simulink model "sampleModel2403_pp_1_1_difftest_difftest"  (R2018a)
settings: Solver=VariableStepAuto  StartTime=0.0  StopTime=10.0  RelTol=1e-3
undefined symbols (not defined in the file): DiscIntNeverNeededParam, sigbuilder_block
libraries: simulink x106
(part 2 of 2)

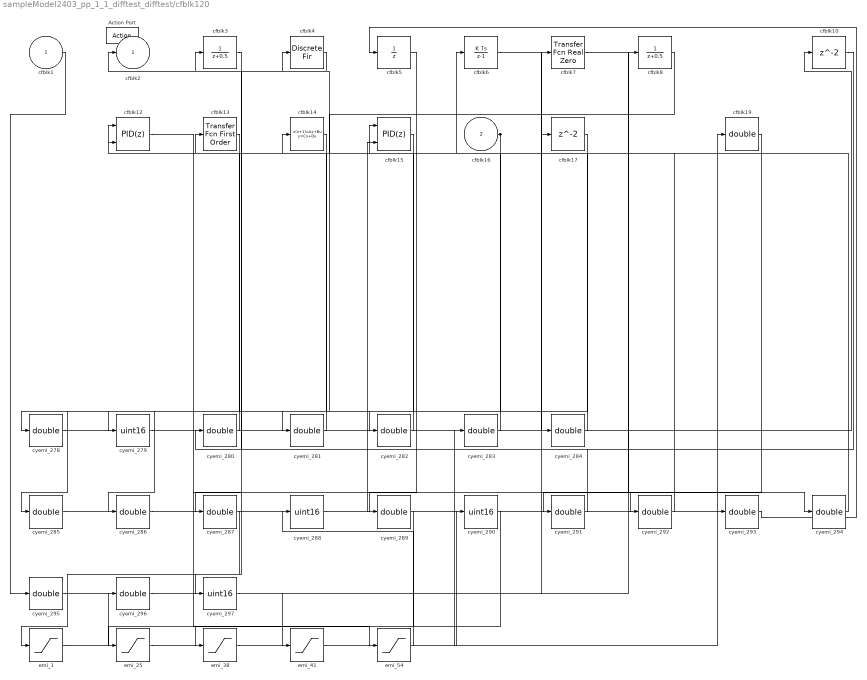
== system sampleModel2403_pp_1_1_difftest_difftest/cfblk120 ==
  cfblk1 : Inport
  cfblk16 : Inport  Port=2
  Action Port : ActionPort  ActionType=then
  cfblk10 : Delay
  cfblk12 : simulink/Continuous/PID Controller (2DOF)  Controller=PID  TimeDomain=Discrete-time  SampleTime=-1  IntegratorMethod=Forward Euler  FilterMethod=Forward Euler  Form=Parallel  UseFilter=on  ControllerParametersSource=internal  P=1  I=1  D=0  N=100  b=1  c=1  InitialConditionSource=internal  InitialConditionForIntegrator=0  InitialConditionForFilter=0  ExternalReset=none  LimitOutput=off  UpperSaturationLimit=inf  LowerSaturationLimit=-inf  LinearizeAsGain=off  AntiWindupMode=none  Kb=1  TrackingMode=off  Kt=1  PParamMin=[]  PParamMax=[]  IParamMin=[]  IParamMax=[]  DParamMin=[]  DParamMax=[]  NParamMin=[]  NParamMax=[]  bParamMin=[]  bParamMax=[]  cParamMin=[]  cParamMax=[]  KbParamMin=[]  KbParamMax=[]  KtParamMin=[]  KtParamMax=[]  POutMin=[]  POutMax=[]  IOutMin=[]  IOutMax=[]  DOutMin=[]  DOutMax=[]  NOutMin=[]  NOutMax=[]  bOutMin=[]  bOutMax=[]  cOutMin=[]  cOutMax=[]  KbOutMin=[]  KbOutMax=[]  KtOutMin=[]  KtOutMax=[]  IntegratorOutMin=[]  IntegratorOutMax=[]  FilterOutMin=[]  FilterOutMax=[]  SumOutMin=[]  SumOutMax=[]  Sum1OutMin=[]  Sum1OutMax=[]  Sum2OutMin=[]  Sum2OutMax=[]  Sum3OutMin=[]  Sum3OutMax=[]  SumI1OutMin=[]  SumI1OutMax=[]  SumI2OutMin=[]  SumI2OutMax=[]  SumI3OutMin=[]  SumI3OutMax=[]  SumDOutMin=[]  SumDOutMax=[]  SaturationOutMin=[]  SaturationOutMax=[]  IntegratorContinuousStateAttributes=''  IntegratorStateMustResolveToSignalObject=off  IntegratorRTWStateStorageClass=Auto  FilterContinuousStateAttributes=''  FilterStateMustResolveToSignalObject=off  FilterRTWStateStorageClass=Auto  DifferentiatorICPrevScaledInput=0  DifferentiatorOutMin=[]  DifferentiatorOutMax=[]  FilterDiffOutCoefMin=[]  FilterDiffOutCoefMax=[]  SumDenOutMin=[]  SumDenOutMax=[]  SumNumOutMin=[]  SumNumOutMax=[]  ReciprocalOutMin=[]  ReciprocalOutMax=[]  DivideOutMin=[]  DivideOutMax=[]  TunerSelectOption=Transfer Function Based (PID Tuner App)
  cfblk13 : simulink/Discrete/Transfer Fcn First Order  PoleZ=0.95  ICPrevOutput=0.0  DoSatur=off
      settings: SourceProductName=Simulink
  cfblk14 : DiscreteStateSpace  SampleTime=-1
  cfblk15 : simulink/Continuous/PID Controller (2DOF)  Controller=PID  TimeDomain=Discrete-time  SampleTime=-1  IntegratorMethod=Forward Euler  FilterMethod=Forward Euler  Form=Parallel  UseFilter=on  ControllerParametersSource=internal  P=1  I=1  D=0  N=100  b=1  c=1  InitialConditionSource=internal  InitialConditionForIntegrator=0  InitialConditionForFilter=0  ExternalReset=none  LimitOutput=off  UpperSaturationLimit=inf  LowerSaturationLimit=-inf  LinearizeAsGain=off  AntiWindupMode=none  Kb=1  TrackingMode=off  Kt=1  PParamMin=[]  PParamMax=[]  IParamMin=[]  IParamMax=[]  DParamMin=[]  DParamMax=[]  NParamMin=[]  NParamMax=[]  bParamMin=[]  bParamMax=[]  cParamMin=[]  cParamMax=[]  KbParamMin=[]  KbParamMax=[]  KtParamMin=[]  KtParamMax=[]  POutMin=[]  POutMax=[]  IOutMin=[]  IOutMax=[]  DOutMin=[]  DOutMax=[]  NOutMin=[]  NOutMax=[]  bOutMin=[]  bOutMax=[]  cOutMin=[]  cOutMax=[]  KbOutMin=[]  KbOutMax=[]  KtOutMin=[]  KtOutMax=[]  IntegratorOutMin=[]  IntegratorOutMax=[]  FilterOutMin=[]  FilterOutMax=[]  SumOutMin=[]  SumOutMax=[]  Sum1OutMin=[]  Sum1OutMax=[]  Sum2OutMin=[]  Sum2OutMax=[]  Sum3OutMin=[]  Sum3OutMax=[]  SumI1OutMin=[]  SumI1OutMax=[]  SumI2OutMin=[]  SumI2OutMax=[]  SumI3OutMin=[]  SumI3OutMax=[]  SumDOutMin=[]  SumDOutMax=[]  SaturationOutMin=[]  SaturationOutMax=[]  IntegratorContinuousStateAttributes=''  IntegratorStateMustResolveToSignalObject=off  IntegratorRTWStateStorageClass=Auto  FilterContinuousStateAttributes=''  FilterStateMustResolveToSignalObject=off  FilterRTWStateStorageClass=Auto  DifferentiatorICPrevScaledInput=0  DifferentiatorOutMin=[]  DifferentiatorOutMax=[]  FilterDiffOutCoefMin=[]  FilterDiffOutCoefMax=[]  SumDenOutMin=[]  SumDenOutMax=[]  SumNumOutMin=[]  SumNumOutMax=[]  ReciprocalOutMin=[]  ReciprocalOutMax=[]  DivideOutMin=[]  DivideOutMax=[]  TunerSelectOption=Transfer Function Based (PID Tuner App)
  cfblk17 : Delay
  cfblk19 : DataTypeConversion  OutDataTypeStr=double
  cfblk3 : DiscreteTransferFcn
  cfblk4 : DiscreteFir
  cfblk5 : UnitDelay  SampleTime=-1
  cfblk6 : DiscreteIntegrator  SampleTime=-1  OutDataTypeStr=double  ICPrevOutput=DiscIntNeverNeededParam  ICPrevScaledInput=DiscIntNeverNeededParam
  cfblk7 : simulink/Discrete/Transfer Fcn Real Zero  ZeroZ=0.75  ICPrevInput=0.0  DoSatur=off
      settings: SourceProductName=Simulink  SourceProductBaseCode=SL
  cfblk8 : DiscreteTransferFcn
  cyemi_{278,280..287,289,291..296} (16 alike) : DataTypeConversion  OutDataTypeStr=double
  cyemi_{279,288,290,297} (4 alike) : DataTypeConversion  OutDataTypeStr=uint16
  emi_{1,25,38,41,54} (5 alike) : Saturate  UpperLimit=0  LowerLimit=0
  cfblk2 : Outport
  wires:
  cfblk4/1 -> cfblk2/1
  cfblk16/1 -> cyemi_279/1, cyemi_297/1
  cyemi_278/1 -> cfblk10/1
  cfblk14/1 -> cyemi_278/1
  cyemi_280/1 -> cfblk12/1
  cfblk10/1 -> cyemi_280/1
  cyemi_281/1 -> cfblk12/2
  cfblk8/1 -> cyemi_281/1
  cyemi_282/1 -> cfblk13/1
  cfblk15/1 -> cyemi_282/1
  cyemi_283/1 -> cfblk14/1
  cyemi_284/1 -> cfblk15/1
  cfblk6/1 -> cyemi_284/1
  cyemi_285/1 -> cfblk15/2
  cfblk17/1 -> cyemi_285/1
  cyemi_286/1 -> cfblk17/1
  cfblk13/1 -> cyemi_286/1
  cfblk3/1 -> cyemi_287/1
  cyemi_288/1 -> cfblk19/1
  cfblk5/1 -> cyemi_289/1
  cyemi_291/1 -> cfblk3/1
  cfblk19/1 -> cyemi_291/1
  cyemi_292/1 -> cfblk4/1
  cfblk12/1 -> cyemi_292/1
  cyemi_293/1 -> cfblk5/1
  cyemi_294/1 -> cfblk6/1
  cfblk7/1 -> cyemi_294/1
  cyemi_295/1 -> cfblk7/1
  cfblk1/1 -> cyemi_295/1
  cyemi_296/1 -> cfblk8/1
  emi_1/1 -> cyemi_296/1
  cyemi_287/1 -> emi_1/1
  emi_25/1 -> cyemi_293/1
  cyemi_290/1 -> emi_25/1
  emi_38/1 -> cyemi_283/1
  cyemi_289/1 -> emi_38/1
  emi_41/1 -> cyemi_290/1
  cyemi_297/1 -> emi_41/1
  emi_54/1 -> cyemi_288/1
  cyemi_279/1 -> emi_54/1

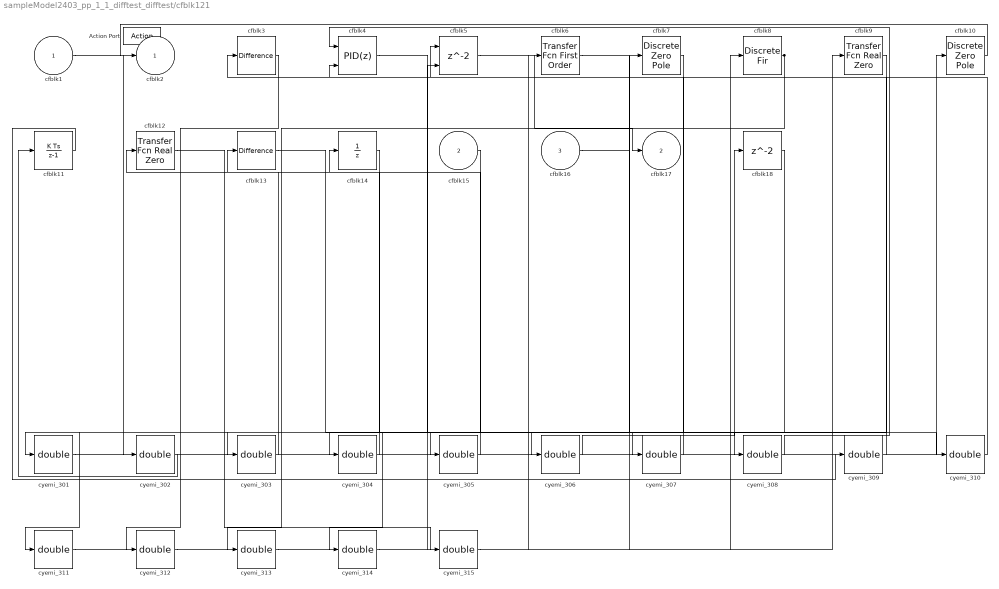
== system sampleModel2403_pp_1_1_difftest_difftest/cfblk121 ==
  cfblk1 : Inport
  cfblk15 : Inport  Port=2
  cfblk16 : Inport  Port=3
  Action Port : ActionPort  ActionType=else
  cfblk10 : DiscreteZeroPole  Poles=[0 0.5]  Gain=1  SampleTime=-1
  cfblk11 : DiscreteIntegrator  SampleTime=-1  OutDataTypeStr=double  ICPrevOutput=DiscIntNeverNeededParam  ICPrevScaledInput=DiscIntNeverNeededParam
  cfblk12 : simulink/Discrete/Transfer Fcn Real Zero  ZeroZ=0.75  ICPrevInput=0.0  DoSatur=off
      settings: SourceProductName=Simulink  SourceProductBaseCode=SL
  cfblk13 : simulink/Discrete/Difference  ICPrevInput=0.0  OutMin=[]  OutMax=[]  OutDataTypeStr=double  OutputDataTypeScalingMode=double  OutDataType=fixdt(1, 16)  OutScaling=2^-10  DoSatur=off
  cfblk14 : UnitDelay  SampleTime=-1
  cfblk18 : Delay
  cfblk3 : simulink/Discrete/Difference  ICPrevInput=0.0  OutMin=[]  OutMax=[]  OutDataTypeStr=double  OutputDataTypeScalingMode=double  OutDataType=fixdt(1, 16)  OutScaling=2^-10  DoSatur=off
  cfblk4 : simulink/Continuous/PID Controller (2DOF)  Controller=PID  TimeDomain=Discrete-time  SampleTime=-1  IntegratorMethod=Forward Euler  FilterMethod=Forward Euler  Form=Parallel  UseFilter=on  ControllerParametersSource=internal  P=1  I=1  D=0  N=100  b=1  c=1  InitialConditionSource=internal  InitialConditionForIntegrator=0  InitialConditionForFilter=0  ExternalReset=none  LimitOutput=off  UpperSaturationLimit=inf  LowerSaturationLimit=-inf  LinearizeAsGain=off  AntiWindupMode=none  Kb=1  TrackingMode=off  Kt=1  PParamMin=[]  PParamMax=[]  IParamMin=[]  IParamMax=[]  DParamMin=[]  DParamMax=[]  NParamMin=[]  NParamMax=[]  bParamMin=[]  bParamMax=[]  cParamMin=[]  cParamMax=[]  KbParamMin=[]  KbParamMax=[]  KtParamMin=[]  KtParamMax=[]  POutMin=[]  POutMax=[]  IOutMin=[]  IOutMax=[]  DOutMin=[]  DOutMax=[]  NOutMin=[]  NOutMax=[]  bOutMin=[]  bOutMax=[]  cOutMin=[]  cOutMax=[]  KbOutMin=[]  KbOutMax=[]  KtOutMin=[]  KtOutMax=[]  IntegratorOutMin=[]  IntegratorOutMax=[]  FilterOutMin=[]  FilterOutMax=[]  SumOutMin=[]  SumOutMax=[]  Sum1OutMin=[]  Sum1OutMax=[]  Sum2OutMin=[]  Sum2OutMax=[]  Sum3OutMin=[]  Sum3OutMax=[]  SumI1OutMin=[]  SumI1OutMax=[]  SumI2OutMin=[]  SumI2OutMax=[]  SumI3OutMin=[]  SumI3OutMax=[]  SumDOutMin=[]  SumDOutMax=[]  SaturationOutMin=[]  SaturationOutMax=[]  IntegratorContinuousStateAttributes=''  IntegratorStateMustResolveToSignalObject=off  IntegratorRTWStateStorageClass=Auto  FilterContinuousStateAttributes=''  FilterStateMustResolveToSignalObject=off  FilterRTWStateStorageClass=Auto  DifferentiatorICPrevScaledInput=0  DifferentiatorOutMin=[]  DifferentiatorOutMax=[]  FilterDiffOutCoefMin=[]  FilterDiffOutCoefMax=[]  SumDenOutMin=[]  SumDenOutMax=[]  SumNumOutMin=[]  SumNumOutMax=[]  ReciprocalOutMin=[]  ReciprocalOutMax=[]  DivideOutMin=[]  DivideOutMax=[]  TunerSelectOption=Transfer Function Based (PID Tuner App)
  cfblk5 : Delay  ShowEnablePort=on
      settings: InputPortMap=u0,e6
  cfblk6 : simulink/Discrete/Transfer Fcn First Order  PoleZ=0.95  ICPrevOutput=0.0  DoSatur=off
      settings: SourceProductName=Simulink
  cfblk7 : DiscreteZeroPole  Poles=[0 0.5]  Gain=1  SampleTime=-1
  cfblk8 : DiscreteFir
  cfblk9 : simulink/Discrete/Transfer Fcn Real Zero  ZeroZ=0.75  ICPrevInput=0.0  DoSatur=off
      settings: SourceProductName=Simulink  SourceProductBaseCode=SL
  cyemi_{301..315} (15 alike) : DataTypeConversion  OutDataTypeStr=double
  cfblk2 : Outport
  cfblk17 : Outport  Port=2
  wires:
  cfblk5/1 -> cfblk17/1
  cfblk8/1 -> cyemi_303/1, cyemi_313/1
  cfblk10/1 -> cfblk2/1
  cyemi_301/1 -> cfblk10/1
  cfblk14/1 -> cyemi_301/1
  cyemi_302/1 -> cfblk11/1
  cfblk1/1 -> cyemi_302/1
  cyemi_303/1 -> cfblk12/1
  cyemi_304/1 -> cfblk13/1
  cfblk7/1 -> cyemi_304/1
  cyemi_305/1 -> cfblk14/1
  cfblk13/1 -> cyemi_305/1
  cyemi_306/1 -> cfblk18/1
  cfblk9/1 -> cyemi_306/1
  cyemi_307/1 -> cfblk3/1
  cfblk4/1 -> cyemi_307/1
  cyemi_308/1 -> cfblk4/1
  cfblk16/1 -> cyemi_308/1
  cyemi_309/1 -> cfblk4/2
  cfblk11/1 -> cyemi_309/1
  cyemi_310/1 -> cfblk5/1
  cfblk6/1 -> cyemi_310/1
  cyemi_311/1 -> cfblk5/2
  cfblk15/1 -> cyemi_311/1
  cyemi_312/1 -> cfblk6/1
  cfblk3/1 -> cyemi_312/1
  cyemi_313/1 -> cfblk7/1
  cyemi_314/1 -> cfblk8/1
  cfblk18/1 -> cyemi_314/1
  cyemi_315/1 -> cfblk9/1
  cfblk12/1 -> cyemi_315/1

== system sampleModel2403_pp_1_1_difftest_difftest/cfblk122 ==
  cfblk1 : Inport
  cfblk10 : Inport  Port=2
  cfblk11 : Inport  Port=3
  Action Port : ActionPort  ActionType=then
  cfblk5 : simulink/Discrete/Transfer Fcn Lead or Lag  PoleZ=0.95  ZeroZ=0.75  ICPrevOutput=0.0  ICPrevInput=0.0  DoSatur=off
      settings: SourceProductName=Simulink  SourceProductBaseCode=SL
  cfblk7 : simulink/Discrete/Transfer Fcn Lead or Lag  PoleZ=0.95  ZeroZ=0.75  ICPrevOutput=0.0  ICPrevInput=0.0  DoSatur=off
      settings: SourceProductName=Simulink  SourceProductBaseCode=SL
  cfblk8 : Delay  ShowEnablePort=on
      settings: InputPortMap=u0,e6
  cyemi_{319..326} (8 alike) : DataTypeConversion  OutDataTypeStr=double
  emi_{11,16,27,48} (4 alike) : Saturate  UpperLimit=0  LowerLimit=0
  cfblk2 : Outport
  cfblk12 : Outport  Port=2
  cfblk13 : Outport  Port=3
  cfblk14 : Outport  Port=4
  wires:
  cfblk5/1 -> cfblk13/1
  cfblk8/1 -> cfblk12/1
  cfblk11/1 -> cfblk2/1, cyemi_320/1
  cfblk1/1 -> cyemi_322/1, cyemi_324/1
  cfblk7/1 -> cfblk14/1
  cyemi_321/1 -> cfblk5/1
  cyemi_323/1 -> cfblk7/1
  cyemi_324/1 -> cfblk8/1
  cyemi_325/1 -> cfblk8/2
  cfblk10/1 -> cyemi_325/1
  emi_11/1 -> cyemi_326/1
  cyemi_319/1 -> emi_11/1
  emi_16/1 -> cyemi_323/1
  cyemi_326/1 -> emi_16/1
  emi_27/1 -> cyemi_321/1
  cyemi_320/1 -> emi_27/1
  emi_48/1 -> cyemi_319/1
  cyemi_322/1 -> emi_48/1

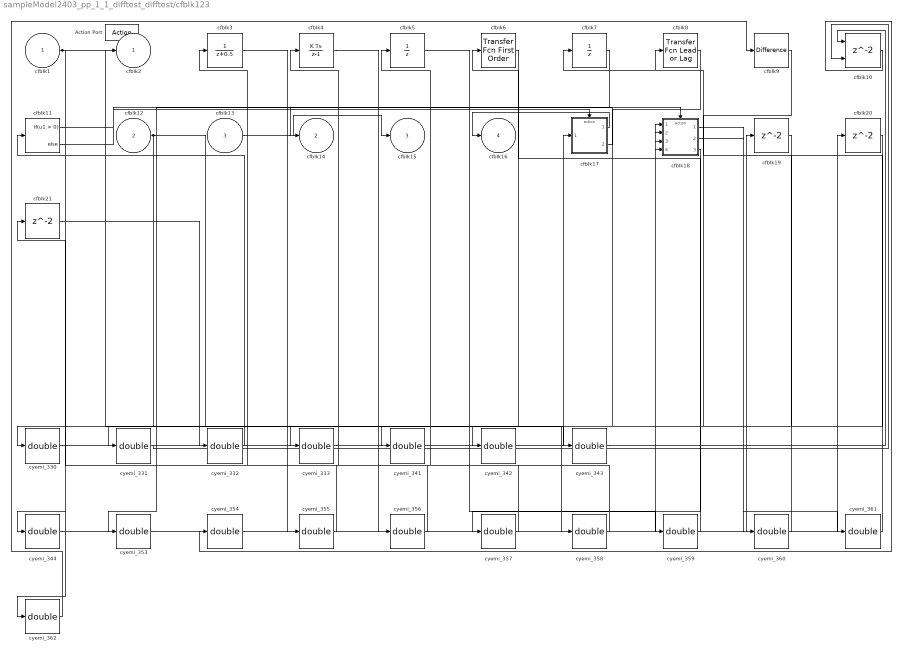
== system sampleModel2403_pp_1_1_difftest_difftest/cfblk123 ==
  cfblk1 : Inport
  cfblk12 : Inport  Port=2
  cfblk13 : Inport  Port=3
  Action Port : ActionPort  ActionType=else
  cfblk10 : Delay  ShowEnablePort=on
      settings: InputPortMap=u0,e6
  cfblk11 : If  SampleTime=1
  cfblk17 : Subsystem  TreatAsAtomicUnit=on
  cfblk18 : Subsystem  TreatAsAtomicUnit=on
  cfblk19 : Delay
  cfblk20 : Delay
  cfblk21 : Delay
  cfblk3 : DiscreteTransferFcn
  cfblk4 : DiscreteIntegrator  SampleTime=-1  OutDataTypeStr=double  ICPrevOutput=DiscIntNeverNeededParam  ICPrevScaledInput=DiscIntNeverNeededParam
  cfblk5 : UnitDelay  SampleTime=-1
  cfblk6 : simulink/Discrete/Transfer Fcn First Order  PoleZ=0.95  ICPrevOutput=0.0  DoSatur=off
      settings: SourceProductName=Simulink
  cfblk7 : UnitDelay  SampleTime=-1
  cfblk8 : simulink/Discrete/Transfer Fcn Lead or Lag  PoleZ=0.95  ZeroZ=0.75  ICPrevOutput=0.0  ICPrevInput=0.0  DoSatur=off
      settings: SourceProductName=Simulink  SourceProductBaseCode=SL
  cfblk9 : simulink/Discrete/Difference  ICPrevInput=0.0  OutMin=[]  OutMax=[]  OutDataTypeStr=double  OutputDataTypeScalingMode=double  OutDataType=fixdt(1, 16)  OutScaling=2^-10  DoSatur=off
  cyemi_{330..333,341..344,353..362} (18 alike) : DataTypeConversion  OutDataTypeStr=double
  cfblk2 : Outport
  cfblk14 : Outport  Port=2
  cfblk15 : Outport  Port=3
  cfblk16 : Outport  Port=4
  wires:
  cfblk13/1 -> cfblk15/1
  cfblk1/1 -> cfblk2/1, cyemi_343/1, cyemi_344/1
  cfblk12/1 -> cyemi_330/1, cyemi_358/1
  cfblk17/1(cfblk2) -> cfblk16/1
  cfblk17/2(cfblk9) -> cfblk14/1
  cfblk11/1 -> cfblk17/Action
  cfblk11/2 -> cfblk18/Action
  cyemi_330/1 -> cfblk10/1
  cyemi_331/1 -> cfblk10/2
  cfblk8/1 -> cyemi_331/1
  cyemi_332/1 -> cfblk11/1
  cfblk21/1 -> cyemi_332/1
  cyemi_333/1 -> cfblk17/1(cfblk1)
  cfblk9/1 -> cyemi_333/1
  cyemi_341/1 -> cfblk18/1(cfblk1)
  cfblk19/1 -> cyemi_341/1
  cyemi_342/1 -> cfblk18/2(cfblk9)
  cfblk20/1 -> cyemi_342/1
  cyemi_343/1 -> cfblk18/3(cfblk10)
  cyemi_344/1 -> cfblk18/4(cfblk11)
  cyemi_353/1 -> cfblk19/1
  cfblk7/1 -> cyemi_353/1
  cyemi_354/1 -> cfblk20/1
  cfblk10/1 -> cyemi_354/1
  cyemi_355/1 -> cfblk21/1
  cfblk3/1 -> cyemi_355/1
  cyemi_356/1 -> cfblk3/1
  cfblk4/1 -> cyemi_356/1
  cyemi_357/1 -> cfblk4/1
  cfblk18/3(cfblk13) -> cyemi_357/1
  cyemi_358/1 -> cfblk5/1
  cyemi_359/1 -> cfblk6/1
  cfblk5/1 -> cyemi_359/1
  cyemi_360/1 -> cfblk7/1
  cfblk18/1(cfblk2) -> cyemi_360/1
  cyemi_361/1 -> cfblk8/1
  cfblk18/2(cfblk12) -> cyemi_361/1
  cyemi_362/1 -> cfblk9/1
  cfblk6/1 -> cyemi_362/1

== system sampleModel2403_pp_1_1_difftest_difftest/cfblk124 ==
  cfblk1 : Inport
  cfblk7 : Inport  Port=2
  Action Port : ActionPort  ActionType=then
  cfblk4 : Delay  ShowEnablePort=on
      settings: InputPortMap=u0,e6
  cfblk5 : DiscreteTransferFcn
  cyemi_{365..369} (5 alike) : DataTypeConversion  OutDataTypeStr=double
  emi_30 : Saturate  UpperLimit=0  LowerLimit=0
  emi_7 : Saturate  UpperLimit=0  LowerLimit=0
  cfblk2 : Outport
  wires:
  cfblk4/1 -> cfblk2/1
  cyemi_366/1 -> cfblk4/1
  cfblk5/1 -> cyemi_366/1
  cyemi_367/1 -> cfblk4/2
  cfblk7/1 -> cyemi_367/1
  cyemi_368/1 -> cfblk5/1
  cfblk1/1 -> cyemi_369/1
  emi_7/1 -> cyemi_365/1
  cyemi_369/1 -> emi_7/1
  emi_30/1 -> cyemi_368/1
  cyemi_365/1 -> emi_30/1

== system sampleModel2403_pp_1_1_difftest_difftest/cfblk125 ==
  cfblk1 : Inport
  cfblk11 : Inport  Port=2
  cfblk12 : Inport  Port=3
  Action Port : ActionPort  ActionType=else
  cfblk10 : If  SampleTime=1
  cfblk14 : Subsystem  TreatAsAtomicUnit=on
  cfblk15 : Subsystem  TreatAsAtomicUnit=on
  cfblk3 : simulink/Discrete/Transfer Fcn Real Zero  ZeroZ=0.75  ICPrevInput=0.0  DoSatur=off
      settings: SourceProductName=Simulink  SourceProductBaseCode=SL
  cfblk4 : simulink/Continuous/PID Controller  Controller=PID  TimeDomain=Discrete-time  SampleTime=-1  IntegratorMethod=Forward Euler  FilterMethod=Forward Euler  Form=Parallel  UseFilter=on  ControllerParametersSource=internal  P=1  I=1  D=0  N=100  InitialConditionSource=internal  InitialConditionForIntegrator=0  InitialConditionForFilter=0  ExternalReset=none  LimitOutput=off  UpperSaturationLimit=inf  LowerSaturationLimit=-inf  LinearizeAsGain=off  AntiWindupMode=none  Kb=1  TrackingMode=off  Kt=1  PParamMin=[]  PParamMax=[]  IParamMin=[]  IParamMax=[]  DParamMin=[]  DParamMax=[]  NParamMin=[]  NParamMax=[]  KbParamMin=[]  KbParamMax=[]  KtParamMin=[]  KtParamMax=[]  POutMin=[]  POutMax=[]  IOutMin=[]  IOutMax=[]  DOutMin=[]  DOutMax=[]  NOutMin=[]  NOutMax=[]  KbOutMin=[]  KbOutMax=[]  KtOutMin=[]  KtOutMax=[]  IntegratorOutMin=[]  IntegratorOutMax=[]  FilterOutMin=[]  FilterOutMax=[]  SumOutMin=[]  SumOutMax=[]  SumI1OutMin=[]  SumI1OutMax=[]  SumI2OutMin=[]  SumI2OutMax=[]  SumI3OutMin=[]  SumI3OutMax=[]  SumDOutMin=[]  SumDOutMax=[]  SaturationOutMin=[]  SaturationOutMax=[]  IntegratorContinuousStateAttributes=''  IntegratorStateMustResolveToSignalObject=off  IntegratorRTWStateStorageClass=Auto  FilterContinuousStateAttributes=''  FilterStateMustResolveToSignalObject=off  FilterRTWStateStorageClass=Auto  DifferentiatorICPrevScaledInput=0  DifferentiatorOutMin=[]  DifferentiatorOutMax=[]  FilterDiffOutCoefMin=[]  FilterDiffOutCoefMax=[]  SumDenOutMin=[]  SumDenOutMax=[]  SumNumOutMin=[]  SumNumOutMax=[]  ReciprocalOutMin=[]  ReciprocalOutMax=[]  DivideOutMin=[]  DivideOutMax=[]  TunerSelectOption=Transfer Function Based (PID Tuner App)
  cfblk5 : simulink/Discrete/Transfer Fcn Real Zero  ZeroZ=0.75  ICPrevInput=0.0  DoSatur=off
      settings: SourceProductName=Simulink  SourceProductBaseCode=SL
  cfblk6 : Delay
  cfblk7 : DiscreteFir
  cfblk8 : simulink/Discrete/Transfer Fcn Real Zero  ZeroZ=0.75  ICPrevInput=0.0  DoSatur=off
      settings: SourceProductName=Simulink  SourceProductBaseCode=SL
  cfblk9 : DiscreteFilter
  cyemi_{373..375,387,395..401} (11 alike) : DataTypeConversion  OutDataTypeStr=double
  cfblk2 : Outport
  cfblk13 : Outport  Port=2
  wires:
  cfblk4/1 -> cfblk2/1
  cfblk8/1 -> cfblk13/1
  cfblk10/1 -> cfblk14/Action
  cfblk10/2 -> cfblk15/Action
  cyemi_373/1 -> cfblk10/1
  cfblk5/1 -> cyemi_373/1
  cyemi_374/1 -> cfblk14/1(cfblk1)
  cfblk6/1 -> cyemi_374/1
  cyemi_375/1 -> cfblk14/2(cfblk11)
  cfblk15/1(cfblk2) -> cyemi_375/1
  cyemi_387/1 -> cfblk15/1(cfblk1)
  cfblk3/1 -> cyemi_387/1
  cyemi_395/1 -> cfblk3/1
  cfblk12/1 -> cyemi_395/1
  cyemi_396/1 -> cfblk4/1
  cfblk7/1 -> cyemi_396/1
  cyemi_397/1 -> cfblk5/1
  cfblk11/1 -> cyemi_397/1
  cyemi_398/1 -> cfblk6/1
  cfblk1/1 -> cyemi_398/1
  cyemi_399/1 -> cfblk7/1
  cfblk9/1 -> cyemi_399/1
  cyemi_400/1 -> cfblk8/1
  cfblk14/2(cfblk12) -> cyemi_400/1
  cyemi_401/1 -> cfblk9/1
  cfblk14/1(cfblk2) -> cyemi_401/1

== system sampleModel2403_pp_1_1_difftest_difftest/cfblk87 ==
  Demux : Demux  Tag=STV Demux  Outputs=1
  FromWs : FromWorkspace  Tag=STV FromWs  VariableName=tuvar  SampleTime=0
      SigBuilderData=|
      | common.afterFinalStr = 'Extrapolate'
      | common.sampleTime = 0
      | dataSet.timeRange = [0 10]
      | dataSet.name = 'Group 1'
      | sbobj.Groups.Name = 'Group 1'
      | sbobj.Groups.Signals.Name = 'Signal 1'
      | sbobj.Groups.Signals.XData = [0 4 4 6 6 10]
      | sbobj.Groups.Signals.YData = [0 0 1 1 0 0]
  Signal 1 : Outport  Tag=STV Outport
  wires:
  Demux/1 -> Signal 1/1
  FromWs/1 -> Demux/1

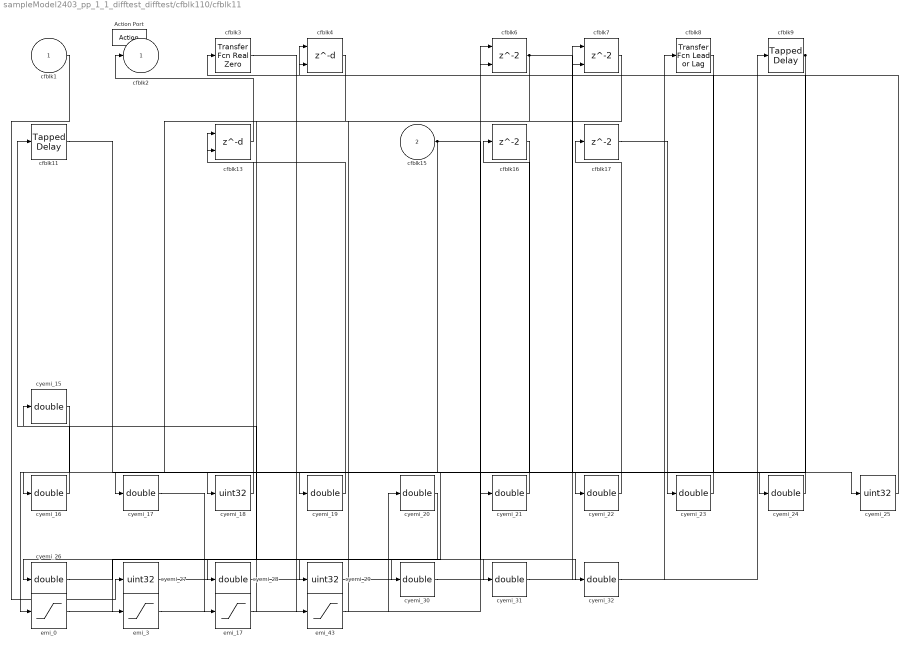
== system sampleModel2403_pp_1_1_difftest_difftest/cfblk110/cfblk11 ==
  cfblk1 : Inport
  cfblk15 : Inport  Port=2
  Action Port : ActionPort  ActionType=then
  cfblk11 : simulink/Discrete/Tapped Delay  vinit=0.0  samptime=-1  NumDelays=1  DelayOrder=Oldest  includeCurrent=off
  cfblk13 : Delay  DelayLengthSource=Input port
      settings: InputPortMap=u0,p1
  cfblk16 : Delay
  cfblk17 : Delay
  cfblk3 : simulink/Discrete/Transfer Fcn Real Zero  ZeroZ=0.75  ICPrevInput=0.0  DoSatur=off
      settings: SourceProductName=Simulink  SourceProductBaseCode=SL
  cfblk4 : Delay  DelayLengthSource=Input port
      settings: InputPortMap=u0,p1
  cfblk6 : Delay  ShowEnablePort=on
      settings: InputPortMap=u0,e6
  cfblk7 : Delay  ShowEnablePort=on
      settings: InputPortMap=u0,e6
  cfblk8 : simulink/Discrete/Transfer Fcn Lead or Lag  PoleZ=0.95  ZeroZ=0.75  ICPrevOutput=0.0  ICPrevInput=0.0  DoSatur=off
      settings: SourceProductName=Simulink  SourceProductBaseCode=SL
  cfblk9 : simulink/Discrete/Tapped Delay  vinit=0.0  samptime=-1  NumDelays=1  DelayOrder=Oldest  includeCurrent=off
  cyemi_{15..17,19..24,26,28,30..32} (14 alike) : DataTypeConversion  OutDataTypeStr=double
  cyemi_{18,25,27,29} (4 alike) : DataTypeConversion  OutDataTypeStr=uint32
  emi_{0,3,17,43} (4 alike) : Saturate  UpperLimit=0  LowerLimit=0
  cfblk2 : Outport
  wires:
  cfblk9/1 -> cyemi_24/1, cyemi_30/1
  cfblk15/1 -> cyemi_19/1, cyemi_32/1
  cfblk13/1 -> cfblk2/1
  cfblk6/1 -> cyemi_25/1, cyemi_29/1
  cyemi_16/1 -> cfblk11/1
  cfblk8/1 -> cyemi_16/1
  cfblk4/1 -> cyemi_17/1
  cyemi_18/1 -> cfblk13/1
  cfblk7/1 -> cyemi_18/1
  cyemi_19/1 -> cfblk13/2
  cyemi_21/1 -> cfblk16/1
  cyemi_22/1 -> cfblk17/1
  cfblk11/1 -> cyemi_22/1
  cyemi_23/1 -> cfblk3/1
  cfblk17/1 -> cyemi_23/1
  cyemi_24/1 -> cfblk4/1
  cyemi_25/1 -> cfblk4/2
  cyemi_27/1 -> cfblk6/1
  cfblk1/1 -> cyemi_27/1
  cyemi_28/1 -> cfblk6/2
  cfblk16/1 -> cyemi_28/1
  cyemi_29/1 -> cfblk7/1
  cyemi_30/1 -> cfblk7/2
  cyemi_31/1 -> cfblk8/1
  cfblk3/1 -> cyemi_31/1
  cyemi_32/1 -> cfblk9/1
  emi_0/1 -> cyemi_20/1
  cyemi_15/1 -> emi_0/1
  emi_3/1 -> cyemi_21/1
  cyemi_20/1 -> emi_3/1
  emi_17/1 -> cyemi_15/1
  cyemi_26/1 -> emi_17/1
  emi_43/1 -> cyemi_26/1
  cyemi_17/1 -> emi_43/1

== system sampleModel2403_pp_1_1_difftest_difftest/cfblk110/cfblk12 ==
  cfblk1 : Inport
  cfblk7 : Inport  Port=2
  Action Port : ActionPort  ActionType=else
  cfblk3 : DiscreteIntegrator  SampleTime=-1  OutDataTypeStr=uint32  ICPrevOutput=DiscIntNeverNeededParam  ICPrevScaledInput=DiscIntNeverNeededParam
  cfblk4 : simulink/Discrete/Transfer Fcn Real Zero  ZeroZ=0.75  ICPrevInput=0.0  DoSatur=off
      settings: SourceProductName=Simulink  SourceProductBaseCode=SL
  cfblk5 : DiscreteFir
  cfblk6 : simulink/Discrete/Tapped Delay  vinit=0.0  samptime=-1  NumDelays=1  DelayOrder=Oldest  includeCurrent=off
  cyemi_35 : DataTypeConversion  OutDataTypeStr=uint32
  cyemi_36 : DataTypeConversion  OutDataTypeStr=uint32
  cyemi_37 : DataTypeConversion  OutDataTypeStr=double
  cyemi_38 : DataTypeConversion  OutDataTypeStr=uint32
  cfblk2 : Outport
  cfblk8 : Outport  Port=2
  cfblk9 : Outport  Port=3
  wires:
  cfblk7/1 -> cfblk8/1, cyemi_37/1
  cfblk4/1 -> cfblk2/1
  cfblk5/1 -> cfblk9/1
  cyemi_35/1 -> cfblk3/1
  cfblk6/1 -> cyemi_35/1
  cyemi_36/1 -> cfblk4/1
  cfblk3/1 -> cyemi_36/1
  cyemi_37/1 -> cfblk5/1
  cyemi_38/1 -> cfblk6/1
  cfblk1/1 -> cyemi_38/1

== system sampleModel2403_pp_1_1_difftest_difftest/cfblk116/cfblk16 ==
  cfblk1 : Inport
  cfblk6 : Inport  Port=2
  Action Port : ActionPort  ActionType=then
  cfblk3 : DiscreteTransferFcn
  cfblk4 : simulink/Discrete/Transfer Fcn First Order  PoleZ=0.95  ICPrevOutput=0.0  DoSatur=off
      settings: SourceProductName=Simulink
  cfblk5 : DiscreteFir
  cyemi_106 : DataTypeConversion  OutDataTypeStr=double
  cyemi_107 : DataTypeConversion  OutDataTypeStr=double
  cyemi_108 : DataTypeConversion  OutDataTypeStr=double
  cfblk2 : Outport
  cfblk7 : Outport  Port=2
  cfblk8 : Outport  Port=3
  wires:
  cfblk3/1 -> cfblk8/1, cyemi_107/1
  cfblk6/1 -> cfblk7/1
  cfblk5/1 -> cfblk2/1
  cyemi_106/1 -> cfblk3/1
  cfblk1/1 -> cyemi_106/1
  cyemi_107/1 -> cfblk4/1
  cyemi_108/1 -> cfblk5/1
  cfblk4/1 -> cyemi_108/1

== system sampleModel2403_pp_1_1_difftest_difftest/cfblk116/cfblk17 ==
  cfblk1 : Inport
  cfblk8 : Inport  Port=2
  Action Port : ActionPort  ActionType=else
  cfblk3 : DiscreteTransferFcn
  cfblk4 : DiscreteFilter
  cfblk5 : DiscreteZeroPole  Poles=[0 0.5]  Gain=1  SampleTime=-1
  cfblk6 : simulink/Discrete/Transfer Fcn Real Zero  ZeroZ=0.75  ICPrevInput=0.0  DoSatur=off
      settings: SourceProductName=Simulink  SourceProductBaseCode=SL
  cfblk7 : Delay  DelayLengthSource=Input port
      settings: InputPortMap=u0,p1
  cfblk9 : Delay
  cyemi_{111..117} (7 alike) : DataTypeConversion  OutDataTypeStr=double
  cfblk2 : Outport
  wires:
  cfblk4/1 -> cfblk2/1
  cyemi_111/1 -> cfblk3/1
  cfblk7/1 -> cyemi_111/1
  cyemi_112/1 -> cfblk4/1
  cfblk5/1 -> cyemi_112/1
  cyemi_113/1 -> cfblk5/1
  cfblk8/1 -> cyemi_113/1
  cyemi_114/1 -> cfblk6/1
  cfblk1/1 -> cyemi_114/1
  cyemi_115/1 -> cfblk7/1
  cfblk6/1 -> cyemi_115/1
  cyemi_116/1 -> cfblk7/2
  cfblk9/1 -> cyemi_116/1
  cyemi_117/1 -> cfblk9/1
  cfblk3/1 -> cyemi_117/1

== system sampleModel2403_pp_1_1_difftest_difftest/cfblk117/cfblk14 ==
  cfblk1 : Inport
  Action Port : ActionPort  ActionType=then
  cfblk10 : Delay  ShowEnablePort=on
      settings: InputPortMap=u0,e6
  cfblk13 : Delay
  cfblk3 : DiscreteIntegrator  SampleTime=-1  OutDataTypeStr=double  ICPrevOutput=DiscIntNeverNeededParam  ICPrevScaledInput=DiscIntNeverNeededParam
  cfblk4 : simulink/Continuous/PID Controller  Controller=PID  TimeDomain=Discrete-time  SampleTime=-1  IntegratorMethod=Forward Euler  FilterMethod=Forward Euler  Form=Parallel  UseFilter=on  ControllerParametersSource=internal  P=1  I=1  D=0  N=100  InitialConditionSource=internal  InitialConditionForIntegrator=0  InitialConditionForFilter=0  ExternalReset=none  LimitOutput=off  UpperSaturationLimit=inf  LowerSaturationLimit=-inf  LinearizeAsGain=off  AntiWindupMode=none  Kb=1  TrackingMode=off  Kt=1  PParamMin=[]  PParamMax=[]  IParamMin=[]  IParamMax=[]  DParamMin=[]  DParamMax=[]  NParamMin=[]  NParamMax=[]  KbParamMin=[]  KbParamMax=[]  KtParamMin=[]  KtParamMax=[]  POutMin=[]  POutMax=[]  IOutMin=[]  IOutMax=[]  DOutMin=[]  DOutMax=[]  NOutMin=[]  NOutMax=[]  KbOutMin=[]  KbOutMax=[]  KtOutMin=[]  KtOutMax=[]  IntegratorOutMin=[]  IntegratorOutMax=[]  FilterOutMin=[]  FilterOutMax=[]  SumOutMin=[]  SumOutMax=[]  SumI1OutMin=[]  SumI1OutMax=[]  SumI2OutMin=[]  SumI2OutMax=[]  SumI3OutMin=[]  SumI3OutMax=[]  SumDOutMin=[]  SumDOutMax=[]  SaturationOutMin=[]  SaturationOutMax=[]  IntegratorContinuousStateAttributes=''  IntegratorStateMustResolveToSignalObject=off  IntegratorRTWStateStorageClass=Auto  FilterContinuousStateAttributes=''  FilterStateMustResolveToSignalObject=off  FilterRTWStateStorageClass=Auto  DifferentiatorICPrevScaledInput=0  DifferentiatorOutMin=[]  DifferentiatorOutMax=[]  FilterDiffOutCoefMin=[]  FilterDiffOutCoefMax=[]  SumDenOutMin=[]  SumDenOutMax=[]  SumNumOutMin=[]  SumNumOutMax=[]  ReciprocalOutMin=[]  ReciprocalOutMax=[]  DivideOutMin=[]  DivideOutMax=[]  TunerSelectOption=Transfer Function Based (PID Tuner App)
  cfblk5 : DiscreteStateSpace  SampleTime=-1
  cfblk6 : Delay
  cfblk7 : UnitDelay  SampleTime=-1
  cfblk8 : Delay  DelayLengthSource=Input port
      settings: InputPortMap=u0,p1
  cfblk9 : DiscreteFilter
  cyemi_{136..146} (11 alike) : DataTypeConversion  OutDataTypeStr=double
  cfblk2 : Outport
  cfblk11 : Outport  Port=2
  cfblk12 : Outport  Port=3
  wires:
  cfblk7/1 -> cyemi_141/1, cyemi_142/1
  cfblk9/1 -> cfblk11/1, cyemi_140/1
  cfblk3/1 -> cfblk2/1
  cfblk1/1 -> cyemi_137/1, cyemi_144/1
  cfblk10/1 -> cfblk12/1
  cfblk8/1 -> cyemi_143/1, cyemi_146/1
  cyemi_136/1 -> cfblk10/1
  cfblk5/1 -> cyemi_136/1
  cyemi_137/1 -> cfblk10/2
  cyemi_138/1 -> cfblk13/1
  cfblk6/1 -> cyemi_138/1
  cyemi_139/1 -> cfblk3/1
  cfblk4/1 -> cyemi_139/1
  cyemi_140/1 -> cfblk4/1
  cyemi_141/1 -> cfblk5/1
  cyemi_142/1 -> cfblk6/1
  cyemi_143/1 -> cfblk7/1
  cyemi_144/1 -> cfblk8/1
  cyemi_145/1 -> cfblk8/2
  cfblk13/1 -> cyemi_145/1
  cyemi_146/1 -> cfblk9/1

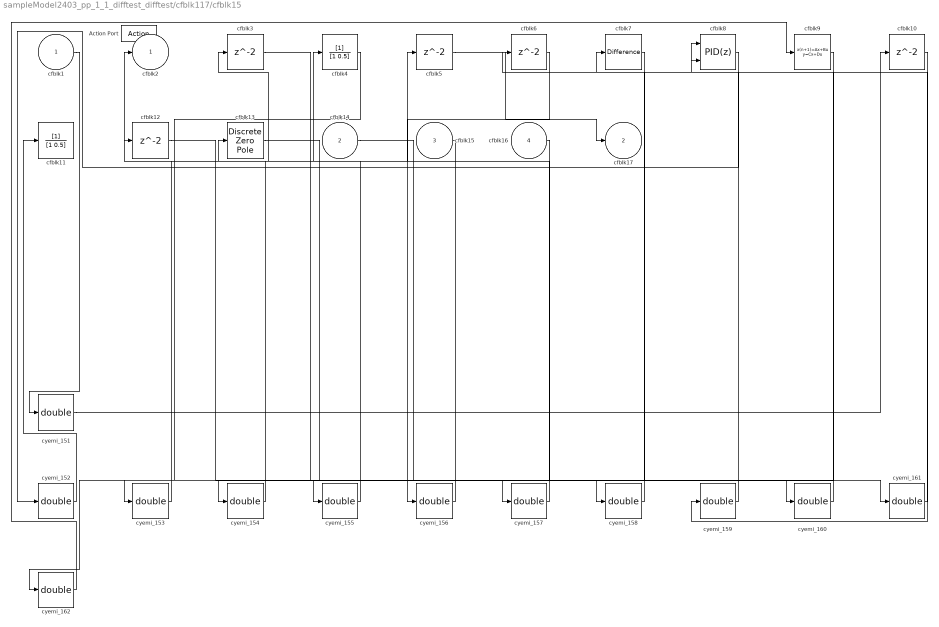
== system sampleModel2403_pp_1_1_difftest_difftest/cfblk117/cfblk15 ==
  cfblk1 : Inport
  cfblk14 : Inport  Port=2
  cfblk15 : Inport  Port=3
  cfblk16 : Inport  Port=4
  Action Port : ActionPort  ActionType=else
  cfblk{3,5..6,10,12} (5 alike) : Delay
  cfblk11 : DiscreteFilter
  cfblk13 : DiscreteZeroPole  Poles=[0 0.5]  Gain=1  SampleTime=-1
  cfblk4 : DiscreteFilter
  cfblk7 : simulink/Discrete/Difference  ICPrevInput=0.0  OutMin=[]  OutMax=[]  OutDataTypeStr=double  OutputDataTypeScalingMode=double  OutDataType=fixdt(1, 16)  OutScaling=2^-10  DoSatur=off
  cfblk8 : simulink/Continuous/PID Controller (2DOF)  Controller=PID  TimeDomain=Discrete-time  SampleTime=-1  IntegratorMethod=Forward Euler  FilterMethod=Forward Euler  Form=Parallel  UseFilter=on  ControllerParametersSource=internal  P=1  I=1  D=0  N=100  b=1  c=1  InitialConditionSource=internal  InitialConditionForIntegrator=0  InitialConditionForFilter=0  ExternalReset=none  LimitOutput=off  UpperSaturationLimit=inf  LowerSaturationLimit=-inf  LinearizeAsGain=off  AntiWindupMode=none  Kb=1  TrackingMode=off  Kt=1  PParamMin=[]  PParamMax=[]  IParamMin=[]  IParamMax=[]  DParamMin=[]  DParamMax=[]  NParamMin=[]  NParamMax=[]  bParamMin=[]  bParamMax=[]  cParamMin=[]  cParamMax=[]  KbParamMin=[]  KbParamMax=[]  KtParamMin=[]  KtParamMax=[]  POutMin=[]  POutMax=[]  IOutMin=[]  IOutMax=[]  DOutMin=[]  DOutMax=[]  NOutMin=[]  NOutMax=[]  bOutMin=[]  bOutMax=[]  cOutMin=[]  cOutMax=[]  KbOutMin=[]  KbOutMax=[]  KtOutMin=[]  KtOutMax=[]  IntegratorOutMin=[]  IntegratorOutMax=[]  FilterOutMin=[]  FilterOutMax=[]  SumOutMin=[]  SumOutMax=[]  Sum1OutMin=[]  Sum1OutMax=[]  Sum2OutMin=[]  Sum2OutMax=[]  Sum3OutMin=[]  Sum3OutMax=[]  SumI1OutMin=[]  SumI1OutMax=[]  SumI2OutMin=[]  SumI2OutMax=[]  SumI3OutMin=[]  SumI3OutMax=[]  SumDOutMin=[]  SumDOutMax=[]  SaturationOutMin=[]  SaturationOutMax=[]  IntegratorContinuousStateAttributes=''  IntegratorStateMustResolveToSignalObject=off  IntegratorRTWStateStorageClass=Auto  FilterContinuousStateAttributes=''  FilterStateMustResolveToSignalObject=off  FilterRTWStateStorageClass=Auto  DifferentiatorICPrevScaledInput=0  DifferentiatorOutMin=[]  DifferentiatorOutMax=[]  FilterDiffOutCoefMin=[]  FilterDiffOutCoefMax=[]  SumDenOutMin=[]  SumDenOutMax=[]  SumNumOutMin=[]  SumNumOutMax=[]  ReciprocalOutMin=[]  ReciprocalOutMax=[]  DivideOutMin=[]  DivideOutMax=[]  TunerSelectOption=Transfer Function Based (PID Tuner App)
  cfblk9 : DiscreteStateSpace  SampleTime=-1
  cyemi_{151..162} (12 alike) : DataTypeConversion  OutDataTypeStr=double
  cfblk2 : Outport
  cfblk17 : Outport  Port=2
  wires:
  cfblk15/1 -> cfblk2/1
  cfblk5/1 -> cfblk17/1
  cyemi_151/1 -> cfblk10/1
  cfblk1/1 -> cyemi_151/1
  cyemi_152/1 -> cfblk11/1
  cfblk8/1 -> cyemi_152/1
  cyemi_153/1 -> cfblk12/1
  cfblk4/1 -> cyemi_153/1
  cyemi_154/1 -> cfblk13/1
  cfblk16/1 -> cyemi_154/1
  cyemi_155/1 -> cfblk3/1
  cfblk12/1 -> cyemi_155/1
  cyemi_156/1 -> cfblk4/1
  cfblk6/1 -> cyemi_156/1
  cyemi_157/1 -> cfblk5/1
  cfblk13/1 -> cyemi_157/1
  cyemi_158/1 -> cfblk6/1
  cfblk9/1 -> cyemi_158/1
  cyemi_159/1 -> cfblk7/1
  cfblk10/1 -> cyemi_159/1
  cyemi_160/1 -> cfblk8/1
  cfblk14/1 -> cyemi_160/1
  cyemi_161/1 -> cfblk8/2
  cfblk3/1 -> cyemi_161/1
  cyemi_162/1 -> cfblk9/1
  cfblk7/1 -> cyemi_162/1

== system sampleModel2403_pp_1_1_difftest_difftest/cfblk117/cfblk16 ==
  cfblk1 : Inport
  cfblk8 : Inport  Port=2
  Action Port : ActionPort  ActionType=then
  cfblk10 : Delay
  cfblk3 : simulink/Discrete/Difference  ICPrevInput=0.0  OutMin=[]  OutMax=[]  OutDataTypeStr=double  OutputDataTypeScalingMode=double  OutDataType=fixdt(1, 16)  OutScaling=2^-10  DoSatur=off
  cfblk6 : simulink/Discrete/Difference  ICPrevInput=0.0  OutMin=[]  OutMax=[]  OutDataTypeStr=double  OutputDataTypeScalingMode=double  OutDataType=fixdt(1, 16)  OutScaling=2^-10  DoSatur=off
  cfblk7 : Delay  DelayLengthSource=Input port
      settings: InputPortMap=u0,p1
  cyemi_{165..171} (7 alike) : DataTypeConversion  OutDataTypeStr=double
  emi_15 : Saturate  UpperLimit=0  LowerLimit=0
  emi_18 : Saturate  UpperLimit=0  LowerLimit=0
  cfblk2 : Outport
  cfblk9 : Outport  Port=2
  wires:
  cfblk8/1 -> cfblk2/1
  cfblk7/1 -> cfblk9/1, cyemi_167/1
  cyemi_165/1 -> cfblk10/1
  cfblk6/1 -> cyemi_165/1
  cyemi_166/1 -> cfblk3/1
  cfblk1/1 -> cyemi_166/1
  cfblk3/1 -> cyemi_168/1
  cyemi_169/1 -> cfblk6/1
  cyemi_170/1 -> cfblk7/1
  cfblk10/1 -> cyemi_170/1
  cyemi_171/1 -> cfblk7/2
  emi_15/1 -> cyemi_171/1
  cyemi_168/1 -> emi_15/1
  emi_18/1 -> cyemi_169/1
  cyemi_167/1 -> emi_18/1

== system sampleModel2403_pp_1_1_difftest_difftest/cfblk117/cfblk17 ==
  cfblk1 : Inport
  Action Port : ActionPort  ActionType=else
  cfblk3 : simulink/Discrete/Transfer Fcn Lead or Lag  PoleZ=0.95  ZeroZ=0.75  ICPrevOutput=0.0  ICPrevInput=0.0  DoSatur=off
      settings: SourceProductName=Simulink  SourceProductBaseCode=SL
  cfblk4 : DiscreteIntegrator  SampleTime=-1  OutDataTypeStr=double  ICPrevOutput=DiscIntNeverNeededParam  ICPrevScaledInput=DiscIntNeverNeededParam
  cfblk5 : Delay
  cfblk6 : DiscreteIntegrator  SampleTime=-1  OutDataTypeStr=double  ICPrevOutput=DiscIntNeverNeededParam  ICPrevScaledInput=DiscIntNeverNeededParam
  cfblk9 : Delay
  cyemi_{173..177} (5 alike) : DataTypeConversion  OutDataTypeStr=double
  cfblk2 : Outport
  cfblk7 : Outport  Port=2
  cfblk8 : Outport  Port=3
  wires:
  cfblk6/1 -> cfblk7/1, cyemi_177/1
  cfblk3/1 -> cfblk2/1
  cfblk5/1 -> cfblk8/1, cyemi_176/1
  cyemi_173/1 -> cfblk3/1
  cfblk4/1 -> cyemi_173/1
  cyemi_174/1 -> cfblk4/1
  cfblk1/1 -> cyemi_174/1
  cyemi_175/1 -> cfblk5/1
  cfblk9/1 -> cyemi_175/1
  cyemi_176/1 -> cfblk6/1
  cyemi_177/1 -> cfblk9/1

== system sampleModel2403_pp_1_1_difftest_difftest/cfblk118/cfblk17 ==
  cfblk1 : Inport
  Action Port : ActionPort  ActionType=then
  cfblk12 : Delay
  cfblk3 : simulink/Discrete/Difference  ICPrevInput=0.0  OutMin=[]  OutMax=[]  OutDataTypeStr=double  OutputDataTypeScalingMode=double  OutDataType=fixdt(1, 16)  OutScaling=2^-10  DoSatur=off
  cfblk4 : simulink/Discrete/Transfer Fcn Lead or Lag  PoleZ=0.95  ZeroZ=0.75  ICPrevOutput=0.0  ICPrevInput=0.0  DoSatur=off
      settings: SourceProductName=Simulink  SourceProductBaseCode=SL
  cfblk6 : simulink/Discrete/Transfer Fcn Lead or Lag  PoleZ=0.95  ZeroZ=0.75  ICPrevOutput=0.0  ICPrevInput=0.0  DoSatur=off
      settings: SourceProductName=Simulink  SourceProductBaseCode=SL
  cfblk7 : Delay  ShowEnablePort=on
      settings: InputPortMap=u0,e6
  cyemi_{203..213} (11 alike) : DataTypeConversion  OutDataTypeStr=double
  emi_{2,37,50,52..53} (5 alike) : Saturate  UpperLimit=0  LowerLimit=0
  cfblk2 : Outport
  cfblk11 : Outport  Port=2
  wires:
  cfblk4/1 -> cfblk11/1
  cfblk1/1 -> cyemi_207/1, cyemi_210/1
  cfblk7/1 -> cyemi_205/1, cyemi_211/1
  cfblk3/1 -> cfblk2/1
  cyemi_204/1 -> cfblk12/1
  cfblk6/1 -> cyemi_204/1
  cyemi_205/1 -> cfblk3/1
  cyemi_206/1 -> cfblk4/1
  cyemi_208/1 -> cfblk6/1
  cyemi_209/1 -> cfblk7/1
  cfblk12/1 -> cyemi_209/1
  cyemi_210/1 -> cfblk7/2
  emi_2/1 -> cyemi_203/1
  cyemi_212/1 -> emi_2/1
  emi_37/1 -> cyemi_212/1
  cyemi_211/1 -> emi_37/1
  emi_50/1 -> cyemi_208/1
  cyemi_203/1 -> emi_50/1
  emi_52/1 -> cyemi_213/1
  cyemi_207/1 -> emi_52/1, emi_53/1
  emi_53/1 -> cyemi_206/1

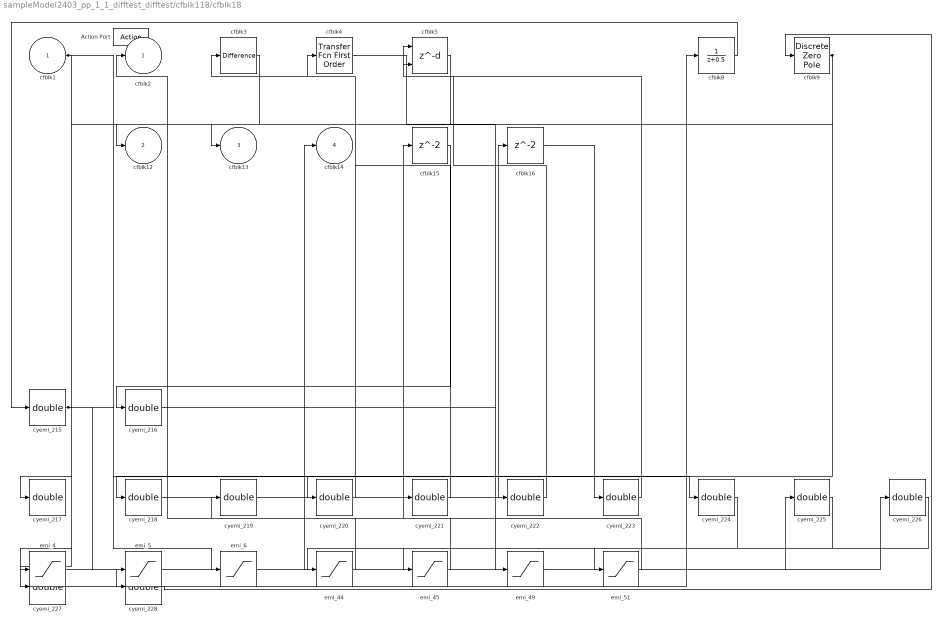
== system sampleModel2403_pp_1_1_difftest_difftest/cfblk118/cfblk18 ==
  cfblk1 : Inport
  Action Port : ActionPort  ActionType=else
  cfblk15 : Delay
  cfblk16 : Delay
  cfblk3 : simulink/Discrete/Difference  ICPrevInput=0.0  OutMin=[]  OutMax=[]  OutDataTypeStr=double  OutputDataTypeScalingMode=double  OutDataType=fixdt(1, 16)  OutScaling=2^-10  DoSatur=off
  cfblk4 : simulink/Discrete/Transfer Fcn First Order  PoleZ=0.95  ICPrevOutput=0.0  DoSatur=off
      settings: SourceProductName=Simulink
  cfblk5 : Delay  DelayLengthSource=Input port
      settings: InputPortMap=u0,p1
  cfblk8 : DiscreteTransferFcn
  cfblk9 : DiscreteZeroPole  Poles=[0 0.5]  Gain=1  SampleTime=-1
  cyemi_{215..228} (14 alike) : DataTypeConversion  OutDataTypeStr=double
  emi_{4..6,44..45,49,51} (7 alike) : Saturate  UpperLimit=0  LowerLimit=0
  cfblk2 : Outport
  cfblk12 : Outport  Port=2
  cfblk13 : Outport  Port=3
  cfblk14 : Outport  Port=4
  wires:
  cfblk9/1 -> cfblk12/1, cyemi_218/1
  cfblk1/1 -> cyemi_217/1, cyemi_220/1, cyemi_224/1
  cfblk3/1 -> cfblk13/1
  cfblk8/1 -> cyemi_215/1
  cfblk15/1 -> cyemi_216/1
  cyemi_218/1 -> cfblk15/1
  cyemi_219/1 -> cfblk16/1
  cyemi_220/1 -> cfblk3/1
  cyemi_221/1 -> cfblk4/1
  cyemi_222/1 -> cfblk5/1
  cfblk4/1 -> cyemi_222/1
  cyemi_223/1 -> cfblk5/2
  cfblk16/1 -> cyemi_223/1
  cyemi_227/1 -> cfblk8/1
  cfblk5/1 -> cyemi_227/1
  cyemi_228/1 -> cfblk9/1
  emi_4/1 -> cyemi_228/1
  cyemi_215/1 -> emi_4/1, emi_5/1, emi_6/1
  emi_5/1 -> cyemi_225/1
  emi_6/1 -> cfblk14/1
  emi_44/1 -> cyemi_219/1
  cyemi_224/1 -> emi_44/1
  emi_45/1 -> cfblk2/1
  cyemi_225/1 -> emi_45/1
  emi_49/1 -> cyemi_226/1
  cyemi_216/1 -> emi_49/1
  emi_51/1 -> cyemi_221/1
  cyemi_226/1 -> emi_51/1

== system sampleModel2403_pp_1_1_difftest_difftest/cfblk118/cfblk19 ==
  cfblk1 : Inport
  Action Port : ActionPort
  cfblk3 : DiscreteIntegrator  SampleTime=-1  OutDataTypeStr=double  ICPrevOutput=DiscIntNeverNeededParam  ICPrevScaledInput=DiscIntNeverNeededParam
  cfblk6 : UnitDelay  SampleTime=-1
  cfblk7 : DiscreteStateSpace  SampleTime=-1
  cyemi_{230..234} (5 alike) : DataTypeConversion  OutDataTypeStr=double
  emi_24 : Saturate  UpperLimit=0  LowerLimit=0
  emi_56 : Saturate  UpperLimit=0  LowerLimit=0
  cfblk2 : Outport
  wires:
  cfblk3/1 -> cfblk2/1
  cyemi_230/1 -> cfblk3/1
  cfblk6/1 -> cyemi_231/1
  cfblk7/1 -> cyemi_232/1
  cyemi_233/1 -> cfblk6/1
  cyemi_234/1 -> cfblk7/1
  cfblk1/1 -> cyemi_234/1
  emi_24/1 -> cyemi_233/1
  cyemi_232/1 -> emi_24/1
  emi_56/1 -> cyemi_230/1
  cyemi_231/1 -> emi_56/1

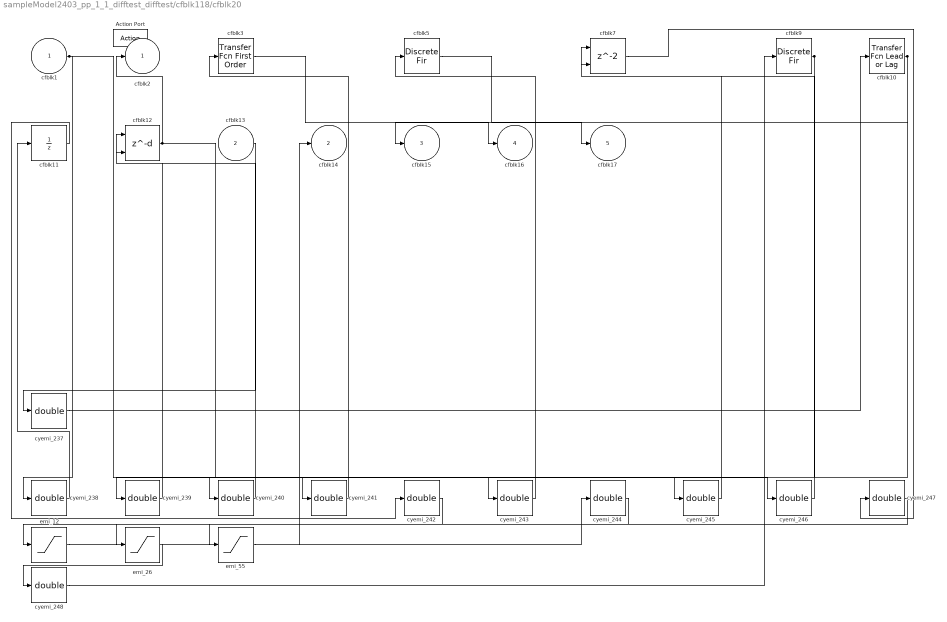
== system sampleModel2403_pp_1_1_difftest_difftest/cfblk118/cfblk20 ==
  cfblk1 : Inport
  cfblk13 : Inport  Port=2
  Action Port : ActionPort
  cfblk10 : simulink/Discrete/Transfer Fcn Lead or Lag  PoleZ=0.95  ZeroZ=0.75  ICPrevOutput=0.0  ICPrevInput=0.0  DoSatur=off
      settings: SourceProductName=Simulink  SourceProductBaseCode=SL
  cfblk11 : UnitDelay  SampleTime=-1
  cfblk12 : Delay  DelayLengthSource=Input port
      settings: InputPortMap=u0,p1
  cfblk3 : simulink/Discrete/Transfer Fcn First Order  PoleZ=0.95  ICPrevOutput=0.0  DoSatur=off
      settings: SourceProductName=Simulink
  cfblk5 : DiscreteFir
  cfblk7 : Delay  ShowEnablePort=on
      settings: InputPortMap=u0,e6
  cfblk9 : DiscreteFir
  cyemi_{237..248} (12 alike) : DataTypeConversion  OutDataTypeStr=double
  emi_12 : Saturate  UpperLimit=0  LowerLimit=0
  emi_26 : Saturate  UpperLimit=0  LowerLimit=0
  emi_55 : Saturate  UpperLimit=0  LowerLimit=0
  cfblk2 : Outport
  cfblk14 : Outport  Port=2
  cfblk15 : Outport  Port=3
  cfblk16 : Outport  Port=4
  cfblk17 : Outport  Port=5
  wires:
  cfblk12/1 -> cfblk2/1, cyemi_243/1
  cfblk5/1 -> cfblk17/1
  cfblk3/1 -> cfblk16/1
  cfblk9/1 -> cyemi_239/1, cyemi_240/1, cyemi_241/1
  cfblk10/1 -> cfblk15/1, cyemi_245/1
  cfblk1/1 -> cyemi_238/1, cyemi_246/1
  cyemi_237/1 -> cfblk10/1
  cfblk13/1 -> cyemi_237/1
  cyemi_238/1 -> cfblk11/1
  cyemi_239/1 -> cfblk12/1
  cyemi_240/1 -> cfblk12/2
  cyemi_241/1 -> cfblk3/1
  cfblk11/1 -> cyemi_242/1
  cyemi_243/1 -> cfblk5/1
  cyemi_245/1 -> cfblk7/1
  cyemi_246/1 -> cfblk7/2
  cfblk7/1 -> cyemi_247/1
  cyemi_248/1 -> cfblk9/1
  emi_12/1 -> cyemi_244/1
  cyemi_242/1 -> emi_12/1
  emi_26/1 -> cyemi_248/1
  cyemi_247/1 -> emi_26/1
  emi_55/1 -> cfblk14/1
  cyemi_244/1 -> emi_55/1

== system sampleModel2403_pp_1_1_difftest_difftest/cfblk123/cfblk17 ==
  cfblk1 : Inport
  Action Port : ActionPort  ActionType=then
  cfblk10 : Delay
  cfblk4 : UnitDelay  SampleTime=-1
  cfblk5 : simulink/Discrete/Transfer Fcn First Order  PoleZ=0.95  ICPrevOutput=0.0  DoSatur=off
      settings: SourceProductName=Simulink
  cfblk7 : DiscreteStateSpace  SampleTime=-1
  cfblk8 : simulink/Continuous/PID Controller  Controller=PID  TimeDomain=Discrete-time  SampleTime=-1  IntegratorMethod=Forward Euler  FilterMethod=Forward Euler  Form=Parallel  UseFilter=on  ControllerParametersSource=internal  P=1  I=1  D=0  N=100  InitialConditionSource=internal  InitialConditionForIntegrator=0  InitialConditionForFilter=0  ExternalReset=none  LimitOutput=off  UpperSaturationLimit=inf  LowerSaturationLimit=-inf  LinearizeAsGain=off  AntiWindupMode=none  Kb=1  TrackingMode=off  Kt=1  PParamMin=[]  PParamMax=[]  IParamMin=[]  IParamMax=[]  DParamMin=[]  DParamMax=[]  NParamMin=[]  NParamMax=[]  KbParamMin=[]  KbParamMax=[]  KtParamMin=[]  KtParamMax=[]  POutMin=[]  POutMax=[]  IOutMin=[]  IOutMax=[]  DOutMin=[]  DOutMax=[]  NOutMin=[]  NOutMax=[]  KbOutMin=[]  KbOutMax=[]  KtOutMin=[]  KtOutMax=[]  IntegratorOutMin=[]  IntegratorOutMax=[]  FilterOutMin=[]  FilterOutMax=[]  SumOutMin=[]  SumOutMax=[]  SumI1OutMin=[]  SumI1OutMax=[]  SumI2OutMin=[]  SumI2OutMax=[]  SumI3OutMin=[]  SumI3OutMax=[]  SumDOutMin=[]  SumDOutMax=[]  SaturationOutMin=[]  SaturationOutMax=[]  IntegratorContinuousStateAttributes=''  IntegratorStateMustResolveToSignalObject=off  IntegratorRTWStateStorageClass=Auto  FilterContinuousStateAttributes=''  FilterStateMustResolveToSignalObject=off  FilterRTWStateStorageClass=Auto  DifferentiatorICPrevScaledInput=0  DifferentiatorOutMin=[]  DifferentiatorOutMax=[]  FilterDiffOutCoefMin=[]  FilterDiffOutCoefMax=[]  SumDenOutMin=[]  SumDenOutMax=[]  SumNumOutMin=[]  SumNumOutMax=[]  ReciprocalOutMin=[]  ReciprocalOutMax=[]  DivideOutMin=[]  DivideOutMax=[]  TunerSelectOption=Transfer Function Based (PID Tuner App)
  cyemi_{334..340} (7 alike) : DataTypeConversion  OutDataTypeStr=double
  emi_28 : Saturate  UpperLimit=0  LowerLimit=0
  emi_29 : Saturate  UpperLimit=0  LowerLimit=0
  emi_46 : Saturate  UpperLimit=0  LowerLimit=0
  cfblk2 : Outport
  cfblk9 : Outport  Port=2
  wires:
  cfblk4/1 -> cfblk2/1
  cfblk8/1 -> cfblk9/1
  cyemi_334/1 -> cfblk10/1
  cfblk7/1 -> cyemi_334/1
  cyemi_336/1 -> cfblk4/1
  cfblk1/1 -> cyemi_336/1
  cyemi_337/1 -> cfblk5/1
  cfblk10/1 -> cyemi_338/1
  cyemi_339/1 -> cfblk7/1
  cyemi_340/1 -> cfblk8/1
  cfblk5/1 -> cyemi_340/1
  emi_28/1 -> cyemi_339/1
  cyemi_338/1 -> emi_28/1, emi_29/1
  emi_29/1 -> cyemi_335/1
  emi_46/1 -> cyemi_337/1
  cyemi_335/1 -> emi_46/1

== system sampleModel2403_pp_1_1_difftest_difftest/cfblk123/cfblk18 ==
  cfblk1 : Inport
  cfblk9 : Inport  Port=2
  cfblk10 : Inport  Port=3
  cfblk11 : Inport  Port=4
  Action Port : ActionPort  ActionType=else
  cfblk14 : Delay
  cfblk3 : DiscreteStateSpace  SampleTime=-1
  cfblk4 : DiscreteFir
  cfblk5 : simulink/Discrete/Difference  ICPrevInput=0.0  OutMin=[]  OutMax=[]  OutDataTypeStr=double  OutputDataTypeScalingMode=double  OutDataType=fixdt(1, 16)  OutScaling=2^-10  DoSatur=off
  cfblk6 : DiscreteStateSpace  SampleTime=-1
  cfblk7 : Delay  ShowEnablePort=on
      settings: InputPortMap=u0,e6
  cfblk8 : simulink/Discrete/Difference  ICPrevInput=0.0  OutMin=[]  OutMax=[]  OutDataTypeStr=double  OutputDataTypeScalingMode=double  OutDataType=fixdt(1, 16)  OutScaling=2^-10  DoSatur=off
  cyemi_{345..352} (8 alike) : DataTypeConversion  OutDataTypeStr=double
  cfblk2 : Outport
  cfblk12 : Outport  Port=2
  cfblk13 : Outport  Port=3
  wires:
  cfblk5/1 -> cfblk13/1
  cfblk11/1 -> cfblk2/1
  cfblk6/1 -> cfblk12/1, cyemi_352/1
  cyemi_345/1 -> cfblk14/1
  cfblk7/1 -> cyemi_345/1
  cyemi_346/1 -> cfblk3/1
  cfblk1/1 -> cyemi_346/1
  cyemi_347/1 -> cfblk4/1
  cfblk14/1 -> cyemi_347/1
  cyemi_348/1 -> cfblk5/1
  cfblk9/1 -> cyemi_348/1
  cyemi_349/1 -> cfblk6/1
  cfblk3/1 -> cyemi_349/1
  cyemi_350/1 -> cfblk7/1
  cfblk4/1 -> cyemi_350/1
  cyemi_351/1 -> cfblk7/2
  cfblk10/1 -> cyemi_351/1
  cyemi_352/1 -> cfblk8/1

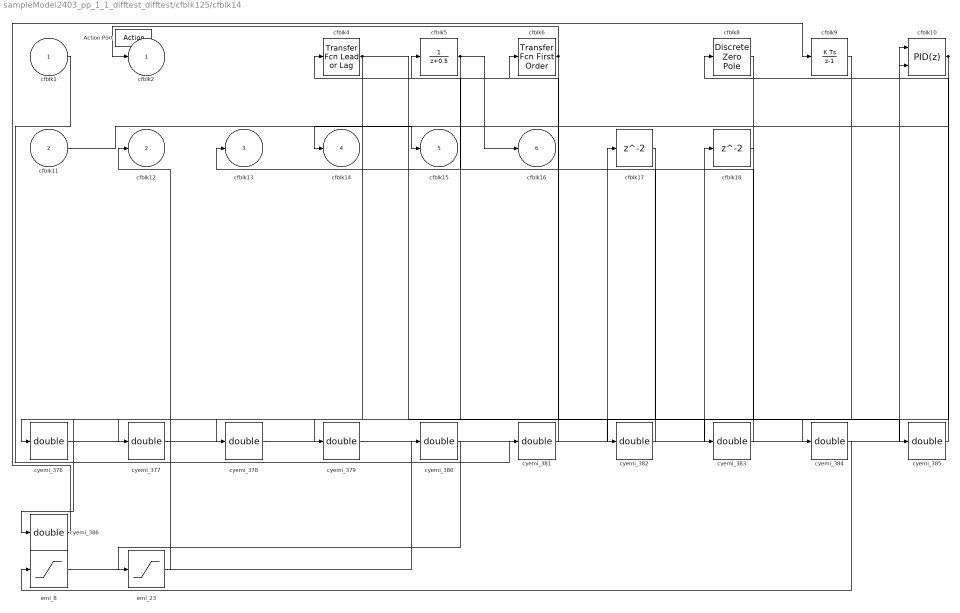
== system sampleModel2403_pp_1_1_difftest_difftest/cfblk125/cfblk14 ==
  cfblk1 : Inport
  cfblk11 : Inport  Port=2
  Action Port : ActionPort  ActionType=then
  cfblk10 : simulink/Continuous/PID Controller (2DOF)  Controller=PID  TimeDomain=Discrete-time  SampleTime=-1  IntegratorMethod=Forward Euler  FilterMethod=Forward Euler  Form=Parallel  UseFilter=on  ControllerParametersSource=internal  P=1  I=1  D=0  N=100  b=1  c=1  InitialConditionSource=internal  InitialConditionForIntegrator=0  InitialConditionForFilter=0  ExternalReset=none  LimitOutput=off  UpperSaturationLimit=inf  LowerSaturationLimit=-inf  LinearizeAsGain=off  AntiWindupMode=none  Kb=1  TrackingMode=off  Kt=1  PParamMin=[]  PParamMax=[]  IParamMin=[]  IParamMax=[]  DParamMin=[]  DParamMax=[]  NParamMin=[]  NParamMax=[]  bParamMin=[]  bParamMax=[]  cParamMin=[]  cParamMax=[]  KbParamMin=[]  KbParamMax=[]  KtParamMin=[]  KtParamMax=[]  POutMin=[]  POutMax=[]  IOutMin=[]  IOutMax=[]  DOutMin=[]  DOutMax=[]  NOutMin=[]  NOutMax=[]  bOutMin=[]  bOutMax=[]  cOutMin=[]  cOutMax=[]  KbOutMin=[]  KbOutMax=[]  KtOutMin=[]  KtOutMax=[]  IntegratorOutMin=[]  IntegratorOutMax=[]  FilterOutMin=[]  FilterOutMax=[]  SumOutMin=[]  SumOutMax=[]  Sum1OutMin=[]  Sum1OutMax=[]  Sum2OutMin=[]  Sum2OutMax=[]  Sum3OutMin=[]  Sum3OutMax=[]  SumI1OutMin=[]  SumI1OutMax=[]  SumI2OutMin=[]  SumI2OutMax=[]  SumI3OutMin=[]  SumI3OutMax=[]  SumDOutMin=[]  SumDOutMax=[]  SaturationOutMin=[]  SaturationOutMax=[]  IntegratorContinuousStateAttributes=''  IntegratorStateMustResolveToSignalObject=off  IntegratorRTWStateStorageClass=Auto  FilterContinuousStateAttributes=''  FilterStateMustResolveToSignalObject=off  FilterRTWStateStorageClass=Auto  DifferentiatorICPrevScaledInput=0  DifferentiatorOutMin=[]  DifferentiatorOutMax=[]  FilterDiffOutCoefMin=[]  FilterDiffOutCoefMax=[]  SumDenOutMin=[]  SumDenOutMax=[]  SumNumOutMin=[]  SumNumOutMax=[]  ReciprocalOutMin=[]  ReciprocalOutMax=[]  DivideOutMin=[]  DivideOutMax=[]  TunerSelectOption=Transfer Function Based (PID Tuner App)
  cfblk17 : Delay
  cfblk18 : Delay
  cfblk4 : simulink/Discrete/Transfer Fcn Lead or Lag  PoleZ=0.95  ZeroZ=0.75  ICPrevOutput=0.0  ICPrevInput=0.0  DoSatur=off
      settings: SourceProductName=Simulink  SourceProductBaseCode=SL
  cfblk5 : DiscreteTransferFcn
  cfblk6 : simulink/Discrete/Transfer Fcn First Order  PoleZ=0.95  ICPrevOutput=0.0  DoSatur=off
      settings: SourceProductName=Simulink
  cfblk8 : DiscreteZeroPole  Poles=[0 0.5]  Gain=1  SampleTime=-1
  cfblk9 : DiscreteIntegrator  SampleTime=-1  OutDataTypeStr=double  ICPrevOutput=DiscIntNeverNeededParam  ICPrevScaledInput=DiscIntNeverNeededParam
  cyemi_{376..386} (11 alike) : DataTypeConversion  OutDataTypeStr=double
  emi_23 : Saturate  UpperLimit=0  LowerLimit=0
  emi_8 : Saturate  UpperLimit=0  LowerLimit=0
  cfblk2 : Outport
  cfblk12 : Outport  Port=2
  cfblk13 : Outport  Port=3
  cfblk14 : Outport  Port=4
  cfblk15 : Outport  Port=5
  cfblk16 : Outport  Port=6
  wires:
  cfblk8/1 -> cfblk13/1
  cfblk11/1 -> cfblk15/1
  cfblk6/1 -> cfblk2/1, cyemi_378/1
  cfblk10/1 -> cfblk14/1, cyemi_379/1, cyemi_383/1
  cfblk5/1 -> cfblk16/1, cyemi_376/1
  cfblk4/1 -> cyemi_385/1, cyemi_386/1
  cyemi_376/1 -> cfblk10/1
  cyemi_377/1 -> cfblk10/2
  cfblk17/1 -> cyemi_377/1
  cyemi_378/1 -> cfblk17/1
  cyemi_379/1 -> cfblk18/1
  cyemi_381/1 -> cfblk4/1
  cfblk1/1 -> cyemi_381/1
  cyemi_382/1 -> cfblk5/1
  cfblk18/1 -> cyemi_382/1
  cyemi_383/1 -> cfblk6/1
  cfblk9/1 -> cyemi_384/1
  cyemi_385/1 -> cfblk8/1
  cyemi_386/1 -> cfblk9/1
  emi_8/1 -> cyemi_380/1
  cyemi_384/1 -> emi_8/1
  emi_23/1 -> cfblk12/1
  cyemi_380/1 -> emi_23/1

== system sampleModel2403_pp_1_1_difftest_difftest/cfblk125/cfblk15 ==
  cfblk1 : Inport
  Action Port : ActionPort  ActionType=else
  cfblk10 : Delay
  cfblk3 : simulink/Continuous/PID Controller  Controller=PID  TimeDomain=Discrete-time  SampleTime=-1  IntegratorMethod=Forward Euler  FilterMethod=Forward Euler  Form=Parallel  UseFilter=on  ControllerParametersSource=internal  P=1  I=1  D=0  N=100  InitialConditionSource=internal  InitialConditionForIntegrator=0  InitialConditionForFilter=0  ExternalReset=none  LimitOutput=off  UpperSaturationLimit=inf  LowerSaturationLimit=-inf  LinearizeAsGain=off  AntiWindupMode=none  Kb=1  TrackingMode=off  Kt=1  PParamMin=[]  PParamMax=[]  IParamMin=[]  IParamMax=[]  DParamMin=[]  DParamMax=[]  NParamMin=[]  NParamMax=[]  KbParamMin=[]  KbParamMax=[]  KtParamMin=[]  KtParamMax=[]  POutMin=[]  POutMax=[]  IOutMin=[]  IOutMax=[]  DOutMin=[]  DOutMax=[]  NOutMin=[]  NOutMax=[]  KbOutMin=[]  KbOutMax=[]  KtOutMin=[]  KtOutMax=[]  IntegratorOutMin=[]  IntegratorOutMax=[]  FilterOutMin=[]  FilterOutMax=[]  SumOutMin=[]  SumOutMax=[]  SumI1OutMin=[]  SumI1OutMax=[]  SumI2OutMin=[]  SumI2OutMax=[]  SumI3OutMin=[]  SumI3OutMax=[]  SumDOutMin=[]  SumDOutMax=[]  SaturationOutMin=[]  SaturationOutMax=[]  IntegratorContinuousStateAttributes=''  IntegratorStateMustResolveToSignalObject=off  IntegratorRTWStateStorageClass=Auto  FilterContinuousStateAttributes=''  FilterStateMustResolveToSignalObject=off  FilterRTWStateStorageClass=Auto  DifferentiatorICPrevScaledInput=0  DifferentiatorOutMin=[]  DifferentiatorOutMax=[]  FilterDiffOutCoefMin=[]  FilterDiffOutCoefMax=[]  SumDenOutMin=[]  SumDenOutMax=[]  SumNumOutMin=[]  SumNumOutMax=[]  ReciprocalOutMin=[]  ReciprocalOutMax=[]  DivideOutMin=[]  DivideOutMax=[]  TunerSelectOption=Transfer Function Based (PID Tuner App)
  cfblk4 : Delay  ShowEnablePort=on
      settings: InputPortMap=u0,e6
  cfblk5 : DiscreteZeroPole  Poles=[0 0.5]  Gain=1  SampleTime=-1
  cfblk6 : DiscreteStateSpace  SampleTime=-1
  cfblk7 : simulink/Discrete/Transfer Fcn Lead or Lag  PoleZ=0.95  ZeroZ=0.75  ICPrevOutput=0.0  ICPrevInput=0.0  DoSatur=off
      settings: SourceProductName=Simulink  SourceProductBaseCode=SL
  cyemi_{388..394} (7 alike) : DataTypeConversion  OutDataTypeStr=double
  cfblk2 : Outport
  cfblk8 : Outport  Port=2
  cfblk9 : Outport  Port=3
  wires:
  cfblk7/1 -> cfblk2/1, cyemi_388/1
  cfblk3/1 -> cfblk9/1, cyemi_392/1
  cfblk4/1 -> cfblk8/1
  cfblk6/1 -> cyemi_391/1, cyemi_394/1
  cyemi_388/1 -> cfblk10/1
  cyemi_389/1 -> cfblk3/1
  cfblk10/1 -> cyemi_389/1
  cyemi_390/1 -> cfblk4/1
  cfblk1/1 -> cyemi_390/1
  cyemi_391/1 -> cfblk4/2
  cyemi_392/1 -> cfblk5/1
  cyemi_393/1 -> cfblk6/1
  cfblk5/1 -> cyemi_393/1
  cyemi_394/1 -> cfblk7/1
